simulink model "ProjectModel23"  (R2023a)
settings: Solver=VariableStepAuto  StartTime=0.0  StopTime=5  RelTol=1e-3
model workspace (MAT data in the model file):
  M = 0.5
  Ts = 0.01
  b = 0.1
  g = 9.8
  l = 0.5
  m = 0.2
settings Model: Creator=sturton  LastModifiedBy=MY PC
settings RTWCC: GPUComputeCapability=5.0

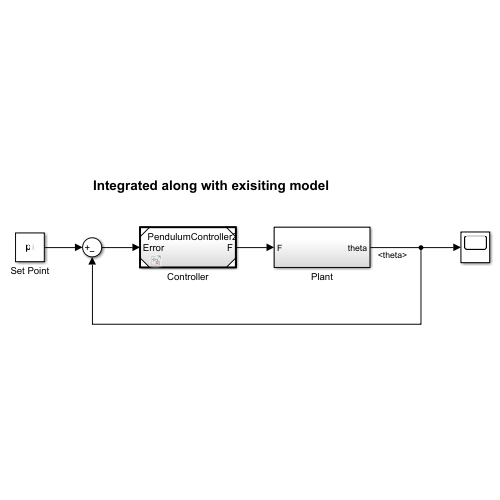
[thumbnail: Simulink's stored preview of the top-level diagram]
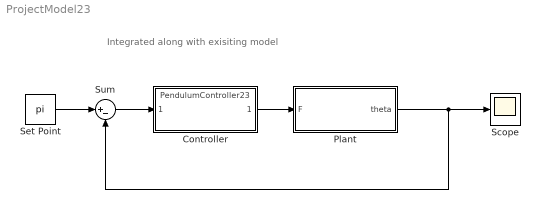
== system ProjectModel23 ==
  note: Integrated along with exisiting model
  Controller : ModelReference  ModelNameDialog=PendulumController23.slx  SimulationMode=Normal  ModelReferenceVersion=1.0
  Plant : Subsystem
  Scope : Scope
  Set Point : Constant  Value=pi
  Sum : Sum  Inputs=|+-
  wires:
  Plant/1(theta) -> Scope/1, Sum/2
  Set Point/1 -> Sum/1
  Sum/1 -> Controller/1
  Controller/1 -> Plant/1(F)

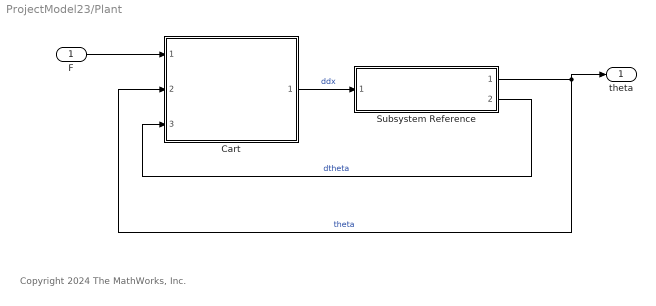
== system ProjectModel23/Plant ==
  note: Copyright 2024 The MathWorks, Inc.
  F : Inport
  Cart : Subsystem  ReferencedSubsystem=CartBase2023a
  Subsystem Reference : Subsystem  ReferencedSubsystem=InvertedPendulum
  theta : Outport
  wires:
  F/1 -> Cart/1
  Cart/1 -> Subsystem Reference/1  "ddx"
  Subsystem Reference/1 -> Cart/2, theta/1  "theta"
  Subsystem Reference/2 -> Cart/3  "dtheta"
